simulink model "Cyber_Physical_Microgrid"  (R2024b)
settings: Solver=VariableStepAuto  StartTime=0.0  StopTime=270  RelTol=1e-3
values from neighbouring files (symbols this model uses):
  Bat =     [initData.mat]
  droopFC1 = 0.05    [initData.mat]
  droopFC2 = 0.05    [initData.mat]
  droopP2 = 0.05    [initData.mat]
  droopQ1 = 0.05    [initData.mat]
  droopQ2 = 0.05    [initData.mat]
  Pref2 = 0.8    [initData.mat]
  Qref1 = 0    [initData.mat]
  Qref2 = 0    [initData.mat]
  timeACLoadCurtail = 200    [initData.mat]
  timeSolarCurtail = 200    [initData.mat]
  Ts = 5e-05    [initData.mat]
  Ts_AC = 0.0002    [initData.mat]
  Ts_DC = 0.001    [initData.mat]
  volt2 = [270.467186401 250.166401688 246.278575679 243.847178474 242.073246789 240.654489675 239.457734124 238.414696845 237.485238449 236.643553985 235.871256975 235.151075236 ... (161 elements, 1x161)]    [initData.mat]
undefined symbols (not defined in the file or in its folder): BattTempBp, CapLUTBp, CapSOCBp, DiscIntNeverNeededParam, Em, Np, Ns, RInt, Tc_Batt
libraries: nesl_utility x55, fl_lib x52, ee_lib x39, modbuslib x16, spsRMSLib x8, simulink x5, spsFourierLib x2, batteryecm_lib x1, eeTransforms x1
(part 3 of 3)

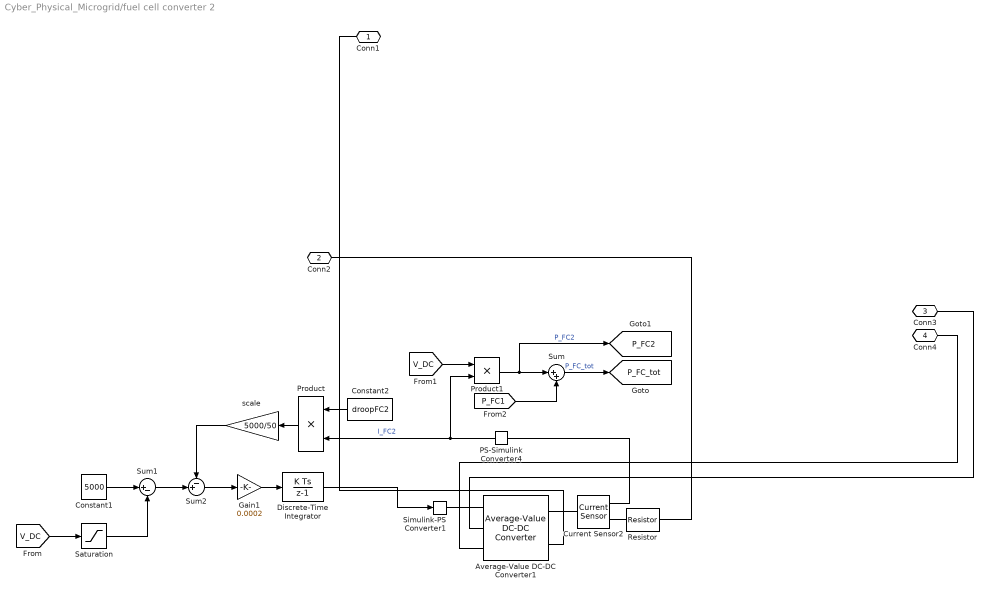
== system Cyber_Physical_Microgrid/fuel cell converter 2 ==
  Average-Value DC-DC Converter1 : ee_lib/Semiconductors & Converters/Converters/Average-Value DC-DC Converter  control_option=ee.enum.converters.controlinput.dutycycle  converter_type=ee.enum.converters.dcdctype.buckboost  efficiency_option=ee.enum.converters.efficiency.constant  efficiency_fixed=100  i_vec=[0, 2, 5] A  efficiency_vec=[90, 95, 98]
      settings: InternalSimscapePortConfiguration="{\"Bottom\":[],\"Left\":[{\"id\":\"DutyCycle\",\"label\":\"DutyCycle\",\"type\":\"input\"},{\"id\":\"p1\",\"label\":\"1+\",\"type\":\"foundation.electrical.electrical\"},{\"id\":\"n1\",\"label\":\"1-\",\"type\":\"foundation.electrical.electrical\"}],\"Right\":[{\"id\":\"p2\",\"label\":\"2+\",\"type\":\"foundation.electrical.electrical\"},{\"id\":\"n2\",\"label\":\"2-\",\"type\":\"foundation.electrical.electrical\"}],\"Top\":[]}"
  Constant1 : Constant  Value=5000  SampleTime=Ts_DC
  Constant2 : Constant  Value=droopFC2  SampleTime=Ts_DC
  Current Sensor2 : fl_lib/Electrical/Electrical Sensors/Current Sensor
  Discrete-Time Integrator : DiscreteIntegrator  InitialCondition=0.5  SampleTime=Ts_DC  LimitOutput=on  UpperSaturationLimit=0.99  LowerSaturationLimit=0  ICPrevOutput=DiscIntNeverNeededParam  ICPrevScaledInput=DiscIntNeverNeededParam
  Gain1 : Gain  Gain=0.0002
  PS-Simulink Converter4 : nesl_utility/PS-Simulink Converter  PhysicalDomain=network_engine_domain  SubClassName=ps_output  LeftPortType=input  RightPortType=output  PseudoPeriodic=off  Frequencies=[]  VectorFormat=1-D array  Unit=inherit  AffineConversion=off
  Product : Product
  Product1 : Product
  Resistor : fl_lib/Electrical/Electrical Elements/Resistor  R=1e-3 Ohm  i_specify=off  i_priority=None  i=0 A  i_nominal_specify=off  i_nominal_value=1  i_nominal_unit=A  v_specify=off  v_priority=None  v=0 V  v_nominal_specify=off  v_nominal_value=1  v_nominal_unit=V
  Saturation : Saturate  UpperLimit=5000
  Simulink-PS Converter1 : nesl_utility/Simulink-PS Converter  PhysicalDomain=network_engine_domain  SubClassName=ps_input  LeftPortType=input  RightPortType=output  PseudoPeriodic=off  Frequencies=[]  NoiseDistribution=none  NoiseParameters=[]  Unit=1  AffineConversion=off  FilteringAndDerivatives=provide  SimscapeFilterOrder=1  InputFilterTimeConstant=0.001  UdotUserProvided=0
  Sum : Sum  Inputs=|++
  Sum1 : Sum  Inputs=|+-
  Sum2 : Sum  Inputs=-+|
  scale : Gain  Gain=5000/50
  Conn1 : PMIOPort  Side=Right
  Conn2 : PMIOPort  Port=2  Side=Right
  Conn3 : PMIOPort  Port=3  Side=Left
  Conn4 : PMIOPort  Port=4  Side=Left
  tag scope: P_FC2=global, P_FC_tot=global
  wires:
  Sum/1 -> [P_FC_tot]  "P_FC_tot"
  Sum1/1 -> Sum2/2
  Product1/1 -> [P_FC2], Sum/1  "P_FC2"
  [P_FC1] -> Sum/2
  [V_DC] -> Product1/1
  Product/1 -> scale/1
  Discrete-Time Integrator/1 -> Simulink-PS Converter1/1
  Gain1/1 -> Discrete-Time Integrator/1
  PS-Simulink Converter4/1 -> Product/2, Product1/2  "I_FC2"
  scale/1 -> Sum2/1
  Constant2/1 -> Product/1
  Saturation/1 -> Sum1/2
  Sum2/1 -> Gain1/1
  Constant1/1 -> Sum1/1
  [V_DC] -> Saturation/1
  connections:
  Current Sensor2/RConn2 -- Resistor/LConn1
  Simulink-PS Converter1/RConn1 -- Average-Value DC-DC Converter1/LConn1
  Conn4/RConn1 -- Average-Value DC-DC Converter1/LConn3
  Conn3/RConn1 -- Average-Value DC-DC Converter1/LConn2
  Current Sensor2/LConn1 -- Average-Value DC-DC Converter1/RConn1
  PS-Simulink Converter4/LConn1 -- Current Sensor2/RConn1
  Average-Value DC-DC Converter1/RConn2 -- Conn1/RConn1
  Resistor/RConn1 -- Conn2/RConn1

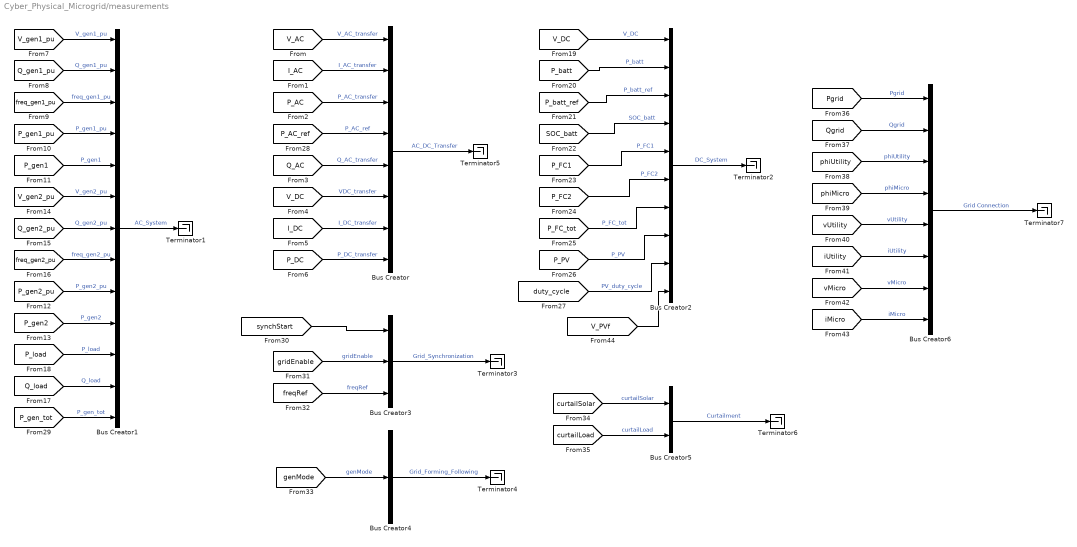
== system Cyber_Physical_Microgrid/measurements ==
  Bus Creator : BusCreator  Inputs=8
  Bus Creator1 : BusCreator  Inputs=13
  Bus Creator2 : BusCreator  Inputs=10
  Bus Creator3 : BusCreator  Inputs=3
  Bus Creator4 : BusCreator  Inputs=1
  Bus Creator5 : BusCreator  Inputs=2
  Bus Creator6 : BusCreator  Inputs=8
  Terminator{1..7} (7 alike) : Terminator
  wires:
  [V_AC] -> Bus Creator/1  "V_AC_transfer"
  [P_AC] -> Bus Creator/3  "P_AC_transfer"
  Bus Creator/1 -> Terminator5/1  "AC_DC_Transfer"
  [I_AC] -> Bus Creator/2  "I_AC_transfer"
  Bus Creator1/1 -> Terminator1/1  "AC_System"
  Bus Creator2/1 -> Terminator2/1  "DC_System"
  [V_gen1_pu] -> Bus Creator1/1  "V_gen1_pu"
  [Q_gen1_pu] -> Bus Creator1/2  "Q_gen1_pu"
  [freq_gen1_pu] -> Bus Creator1/3  "freq_gen1_pu"
  [P_gen1_pu] -> Bus Creator1/4  "P_gen1_pu"
  [P_gen1] -> Bus Creator1/5  "P_gen1"
  [V_gen2_pu] -> Bus Creator1/6  "V_gen2_pu"
  [Q_gen2_pu] -> Bus Creator1/7  "Q_gen2_pu"
  [freq_gen2_pu] -> Bus Creator1/8  "freq_gen2_pu"
  [P_gen2_pu] -> Bus Creator1/9  "P_gen2_pu"
  [P_gen2] -> Bus Creator1/10  "P_gen2"
  [P_load] -> Bus Creator1/11  "P_load"
  [Q_load] -> Bus Creator1/12  "Q_load"
  [V_DC] -> Bus Creator2/1  "V_DC"
  [P_batt] -> Bus Creator2/2  "P_batt"
  [P_batt_ref] -> Bus Creator2/3  "P_batt_ref"
  [SOC_batt] -> Bus Creator2/4  "SOC_batt"
  [P_FC1] -> Bus Creator2/5  "P_FC1"
  [P_FC2] -> Bus Creator2/6  "P_FC2"
  [P_FC_tot] -> Bus Creator2/7  "P_FC_tot"
  [P_PV] -> Bus Creator2/8  "P_PV"
  [duty_cycle] -> Bus Creator2/9  "PV_duty_cycle"
  [P_AC_ref] -> Bus Creator/4  "P_AC_ref"
  [Q_AC] -> Bus Creator/5  "Q_AC_transfer"
  [V_DC] -> Bus Creator/6  "VDC_transfer"
  [I_DC] -> Bus Creator/7  "I_DC_transfer"
  [P_DC] -> Bus Creator/8  "P_DC_transfer"
  [P_gen_tot] -> Bus Creator1/13  "P_gen_tot"
  [gridEnable] -> Bus Creator3/2  "gridEnable"
  Bus Creator3/1 -> Terminator3/1  "Grid_Synchronization"
  [freqRef] -> Bus Creator3/3  "freqRef"
  [genMode] -> Bus Creator4/1  "genMode"
  Bus Creator4/1 -> Terminator4/1  "Grid_Forming_Following"
  Bus Creator5/1 -> Terminator6/1  "Curtailment"
  [curtailLoad] -> Bus Creator5/2  "curtailLoad"
  [curtailSolar] -> Bus Creator5/1  "curtailSolar"
  [Pgrid] -> Bus Creator6/1  "Pgrid"
  [Qgrid] -> Bus Creator6/2  "Qgrid"
  Bus Creator6/1 -> Terminator7/1  "Grid Connection"
  [phiUtility] -> Bus Creator6/3  "phiUtility"
  [phiMicro] -> Bus Creator6/4  "phiMicro"
  [vUtility] -> Bus Creator6/5  "vUtility"
  [iUtility] -> Bus Creator6/6  "iUtility"
  [vMicro] -> Bus Creator6/7  "vMicro"
  [iMicro] -> Bus Creator6/8  "iMicro"
  [synchStart] -> Bus Creator3/1
  [V_PVf] -> Bus Creator2/10

== system Cyber_Physical_Microgrid/ /Form // Follow ==
  note: AVR and exciter control
  genMode : Inport
  Qerror : Inport  Port=2
  Verror : Inport  Port=3
  Constant1 : Constant  Value=500
  Constant2 : Constant  Value=0.5
  Constant3 : Constant  Value=1000
  Constant4 : Constant
  Discrete-Time Integrator : DiscreteIntegrator  gainval=1  InitialCondition=0.1  SampleTime=Ts_AC  ICPrevOutput=DiscIntNeverNeededParam  ICPrevScaledInput=DiscIntNeverNeededParam
  Product : Product
  Product1 : Product
  Sum4 : Sum  Inputs=|++
  Switch : Switch  Criteria=u2 > Threshold  SaturateOnIntegerOverflow=off  InputSameDT=off
  Switch1 : Switch  Criteria=u2 > Threshold  SaturateOnIntegerOverflow=off  InputSameDT=off
  Switch2 : Switch  Criteria=u2 > Threshold  SaturateOnIntegerOverflow=off  InputSameDT=off
  Unit Delay : UnitDelay  SampleTime=Ts_AC  HasFrameUpgradeWarning=on
  T : Outport
  wires:
  Product1/1 -> Unit Delay/1
  genMode/1 -> Switch/2, Switch2/2, Switch1/2
  Constant3/1 -> Switch2/3
  Constant4/1 -> Switch2/1
  Switch2/1 -> Product1/1
  Discrete-Time Integrator/1 -> Sum4/1
  Unit Delay/1 -> Sum4/2
  Constant2/1 -> Switch1/1
  Constant1/1 -> Switch1/3
  Switch/1 -> Product/2, Product1/2
  Product/1 -> Discrete-Time Integrator/1
  Verror/1 -> Switch/3
  Switch1/1 -> Product/1
  Qerror/1 -> Switch/1
  Sum4/1 -> T/1

== system Cyber_Physical_Microgrid/ /Form // Follow1 ==
  note: PRIME MOVER ND GOVRNR CONTROL
  genMode : Inport
  Perror : Inport  Port=2
  Ferror : Inport  Port=3
  Constant1 : Constant  Value=100
  Constant2 : Constant  Value=0.3
  Constant3 : Constant  Value=200
  Constant4 : Constant  Value=0.1
  Discrete-Time Integrator : DiscreteIntegrator  gainval=1  InitialCondition=0.1  SampleTime=Ts_AC  ICPrevOutput=DiscIntNeverNeededParam  ICPrevScaledInput=DiscIntNeverNeededParam
  Product : Product
  Product1 : Product
  Sum4 : Sum  Inputs=|++
  Switch : Switch  Criteria=u2 > Threshold  SaturateOnIntegerOverflow=off  InputSameDT=off
  Switch1 : Switch  Criteria=u2 > Threshold  SaturateOnIntegerOverflow=off  InputSameDT=off
  Switch2 : Switch  Criteria=u2 > Threshold  SaturateOnIntegerOverflow=off  InputSameDT=off
  Unit Delay : UnitDelay  SampleTime=Ts_AC  HasFrameUpgradeWarning=on
  T : Outport
  wires:
  Product1/1 -> Unit Delay/1
  genMode/1 -> Switch/2, Switch2/2, Switch1/2
  Constant3/1 -> Switch2/3
  Constant4/1 -> Switch2/1
  Switch2/1 -> Product1/1
  Discrete-Time Integrator/1 -> Sum4/1
  Unit Delay/1 -> Sum4/2
  Constant2/1 -> Switch1/1
  Constant1/1 -> Switch1/3
  Switch/1 -> Product/2, Product1/2
  Product/1 -> Discrete-Time Integrator/1
  Ferror/1 -> Switch/3
  Switch1/1 -> Product/1
  Perror/1 -> Switch/1
  Sum4/1 -> T/1

== system Cyber_Physical_Microgrid/Generator 02/Form // Follow ==
  genMode : Inport
  Qerror : Inport  Port=2
  Verror : Inport  Port=3
  Constant1 : Constant  Value=500
  Constant2 : Constant  Value=0.5
  Constant3 : Constant  Value=1000
  Constant4 : Constant
  Discrete-Time Integrator : DiscreteIntegrator  gainval=1  InitialCondition=0.1  SampleTime=Ts_AC  ICPrevOutput=DiscIntNeverNeededParam  ICPrevScaledInput=DiscIntNeverNeededParam
  Product : Product
  Product1 : Product
  Sum4 : Sum  Inputs=|++
  Switch : Switch  Criteria=u2 > Threshold  SaturateOnIntegerOverflow=off  InputSameDT=off
  Switch1 : Switch  Criteria=u2 > Threshold  SaturateOnIntegerOverflow=off  InputSameDT=off
  Switch2 : Switch  Criteria=u2 > Threshold  SaturateOnIntegerOverflow=off  InputSameDT=off
  Unit Delay : UnitDelay  SampleTime=Ts_AC  HasFrameUpgradeWarning=on
  T : Outport
  wires:
  Product1/1 -> Unit Delay/1
  genMode/1 -> Switch/2, Switch2/2, Switch1/2
  Constant3/1 -> Switch2/3
  Constant4/1 -> Switch2/1
  Switch2/1 -> Product1/1
  Discrete-Time Integrator/1 -> Sum4/1
  Unit Delay/1 -> Sum4/2
  Constant2/1 -> Switch1/1
  Constant1/1 -> Switch1/3
  Switch/1 -> Product/2, Product1/2
  Product/1 -> Discrete-Time Integrator/1
  Verror/1 -> Switch/3
  Switch1/1 -> Product/1
  Qerror/1 -> Switch/1
  Sum4/1 -> T/1

== system Cyber_Physical_Microgrid/Generator 02/Form // Follow1 ==
  genMode : Inport
  Perror : Inport  Port=2
  Ferror : Inport  Port=3
  Constant1 : Constant  Value=100
  Constant2 : Constant  Value=0.3
  Constant3 : Constant  Value=200
  Constant4 : Constant  Value=0.1
  Discrete-Time Integrator : DiscreteIntegrator  gainval=1  InitialCondition=0.1  SampleTime=Ts_AC  ICPrevOutput=DiscIntNeverNeededParam  ICPrevScaledInput=DiscIntNeverNeededParam
  Product : Product
  Product1 : Product
  Sum4 : Sum  Inputs=|++
  Switch : Switch  Criteria=u2 > Threshold  SaturateOnIntegerOverflow=off  InputSameDT=off
  Switch1 : Switch  Criteria=u2 > Threshold  SaturateOnIntegerOverflow=off  InputSameDT=off
  Switch2 : Switch  Criteria=u2 > Threshold  SaturateOnIntegerOverflow=off  InputSameDT=off
  Unit Delay : UnitDelay  SampleTime=Ts_AC  HasFrameUpgradeWarning=on
  T : Outport
  wires:
  Product1/1 -> Unit Delay/1
  genMode/1 -> Switch/2, Switch2/2, Switch1/2
  Constant3/1 -> Switch2/3
  Constant4/1 -> Switch2/1
  Switch2/1 -> Product1/1
  Discrete-Time Integrator/1 -> Sum4/1
  Unit Delay/1 -> Sum4/2
  Constant2/1 -> Switch1/1
  Constant1/1 -> Switch1/3
  Switch/1 -> Product1/2, Product/2
  Product/1 -> Discrete-Time Integrator/1
  Ferror/1 -> Switch/3
  Switch1/1 -> Product/1
  Perror/1 -> Switch/1
  Sum4/1 -> T/1

== system Cyber_Physical_Microgrid/Generator 02/Subsystem1 ==
  In1 : Inport
  Discrete-Time Integrator : DiscreteIntegrator  gainval=20  SampleTime=Ts_AC  ICPrevOutput=DiscIntNeverNeededParam  ICPrevScaledInput=DiscIntNeverNeededParam
  Sum : Sum  Inputs=|+-
  in1 : Outport
  wires:
  Sum/1 -> Discrete-Time Integrator/1
  Discrete-Time Integrator/1 -> Sum/2, in1/1
  In1/1 -> Sum/1

== system Cyber_Physical_Microgrid/Generator 02/Subsystem2 ==
  In1 : Inport
  Discrete-Time Integrator : DiscreteIntegrator  gainval=20  SampleTime=Ts_AC  ICPrevOutput=DiscIntNeverNeededParam  ICPrevScaledInput=DiscIntNeverNeededParam
  Sum : Sum  Inputs=|+-
  in : Outport
  wires:
  Sum/1 -> Discrete-Time Integrator/1
  Discrete-Time Integrator/1 -> Sum/2, in/1
  In1/1 -> Sum/1

== system Cyber_Physical_Microgrid/PQ meas/Subsystem ==
  In1 : Inport
  Discrete-Time Integrator : DiscreteIntegrator  gainval=20  SampleTime=Ts_AC  ICPrevOutput=DiscIntNeverNeededParam  ICPrevScaledInput=DiscIntNeverNeededParam
  Sum : Sum  Inputs=|+-
  Out1 : Outport
  wires:
  In1/1 -> Sum/1
  Discrete-Time Integrator/1 -> Out1/1, Sum/2
  Sum/1 -> Discrete-Time Integrator/1

== system Cyber_Physical_Microgrid/PQ meas/Subsystem1 ==
  In1 : Inport
  Discrete-Time Integrator : DiscreteIntegrator  gainval=20  SampleTime=Ts_AC  ICPrevOutput=DiscIntNeverNeededParam  ICPrevScaledInput=DiscIntNeverNeededParam
  Sum : Sum  Inputs=|+-
  Out1 : Outport
  wires:
  Sum/1 -> Discrete-Time Integrator/1
  Discrete-Time Integrator/1 -> Sum/2, Out1/1
  In1/1 -> Sum/1

== system Cyber_Physical_Microgrid/PV Array/Sensing Current ==
  Current Sensor : fl_lib/Electrical/Electrical Sensors/Current Sensor
  PS-Simulink/I : nesl_utility/PS-Simulink Converter  PhysicalDomain=network_engine_domain  SubClassName=ps_output  LeftPortType=input  RightPortType=output  PseudoPeriodic=off  Frequencies=[]  VectorFormat=1-D array  Unit=1  AffineConversion=off
  + : PMIOPort  Side=Left
  - : PMIOPort  Port=2  Side=Right
  I : Outport
  wires:
  PS-Simulink/I/1 -> I/1
  connections:
  -/RConn1 -- Current Sensor/RConn2
  Current Sensor/LConn1 -- +/RConn1
  Current Sensor/RConn1 -- PS-Simulink/I/LConn1

== system Cyber_Physical_Microgrid/PV Array/sensing voltage ==
  PS-Simulink Converter : nesl_utility/PS-Simulink Converter  PhysicalDomain=network_engine_domain  SubClassName=ps_output  LeftPortType=input  RightPortType=output  PseudoPeriodic=off  Frequencies=[]  VectorFormat=1-D array  Unit=inherit  AffineConversion=off
  Voltage Sensor : fl_lib/Electrical/Electrical Sensors/Voltage Sensor
  + : PMIOPort  Side=Left
  - : PMIOPort  Port=2  Side=Right
  V : Outport
  wires:
  PS-Simulink Converter/1 -> V/1
  connections:
  Voltage Sensor/LConn1 -- +/RConn1
  Voltage Sensor/RConn2 -- -/RConn1
  Voltage Sensor/RConn1 -- PS-Simulink Converter/LConn1

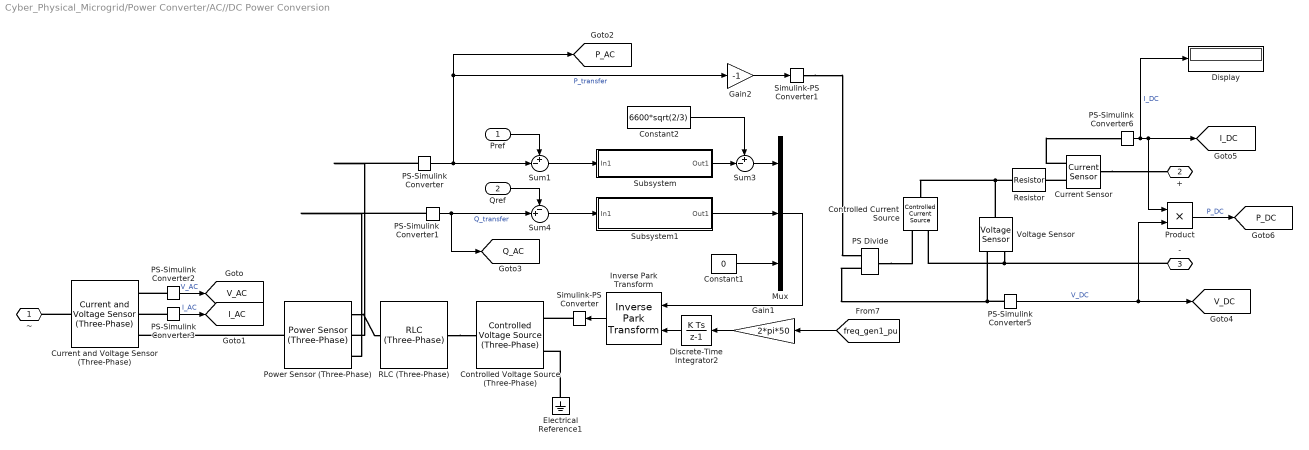
== system Cyber_Physical_Microgrid/Power Converter/AC//DC Power Conversion ==
  Pref : Inport
  Qref : Inport  Port=2
  Constant1 : Constant  Value=0
  Constant2 : Constant  Value=6600*sqrt(2/3)
  Controlled Current Source : fl_lib/Electrical/Electrical Sources/Controlled Current Source
  Controlled Voltage Source (Three-Phase) : ee_lib/Sources/Controlled Voltage Source (Three-Phase)  input_option=ee.enum.inputType.instantaneous  FRated=50 Hz
      settings: InternalSimscapePortConfiguration="{\"Bottom\":[],\"Left\":[{\"id\":\"S\",\"label\":\"S\",\"type\":\"input\"},{\"id\":\"n\",\"label\":\"n\",\"type\":\"foundation.electrical.electrical\"}],\"Right\":[{\"id\":\"N\",\"label\":\"~\",\"type\":\"foundation.electrical.three_phase\"}],\"Top\":[]}"
  Current Sensor : fl_lib/Electrical/Electrical Sensors/Current Sensor
  Current and Voltage Sensor (Three-Phase) : ee_lib/Sensors & Transducers/Current and Voltage Sensor (Three-Phase)  vMeasurementType=ee.enum.vmeasurement.ll  outputUnit=ee.enum.unit.si  SRated=100e6 A*V  VRated=24e3 V  I_specify=off  I_priority=None  I=[0, 0, 0] A  I_nominal_specify=off  I_nominal_value=1  I_nominal_unit=A  V_specify=off  V_priority=None  V=[0, 0, 0] V  V_nominal_specify=off  V_nominal_value=1  V_nominal_unit=V
      settings: InternalSimscapePortConfiguration="{\"Bottom\":[],\"Left\":[{\"id\":\"N1\",\"label\":\"~1\",\"type\":\"foundation.electrical.three_phase\"}],\"Right\":[{\"id\":\"V_output\",\"label\":\"V\",\"type\":\"output\"},{\"id\":\"I_output\",\"label\":\"I\",\"type\":\"output\"},{\"id\":\"N2\",\"label\":\"~2\",\"type\":\"foundation.electrical.three_phase\"}],\"Top\":[]}"
  Discrete-Time Integrator2 : DiscreteIntegrator  SampleTime=Ts_AC  ICPrevOutput=DiscIntNeverNeededParam  ICPrevScaledInput=DiscIntNeverNeededParam
  Display : Display
  Electrical Reference1 : fl_lib/Electrical/Electrical Elements/Electrical Reference
  Gain1 : Gain  Gain=2*pi*50
  Gain2 : Gain  Gain=-1
  Inverse Park Transform : eeTransforms/Inverse Park Transform  AxisAlignment=Q-axis  PowerInvariant=off
  Mux : Mux  Inputs=3
  PS Divide : fl_lib/Physical Signals/Functions/PS Divide
  PS-Simulink Converter : nesl_utility/PS-Simulink Converter  PhysicalDomain=network_engine_domain  SubClassName=ps_output  LeftPortType=input  RightPortType=output  PseudoPeriodic=off  Frequencies=[]  VectorFormat=1-D array  Unit=W  AffineConversion=off
  PS-Simulink Converter1 : nesl_utility/PS-Simulink Converter  PhysicalDomain=network_engine_domain  SubClassName=ps_output  LeftPortType=input  RightPortType=output  PseudoPeriodic=off  Frequencies=[]  VectorFormat=1-D array  Unit=V*A  AffineConversion=off
  PS-Simulink Converter{2..3,5..6} (4 alike) : nesl_utility/PS-Simulink Converter  PhysicalDomain=network_engine_domain  SubClassName=ps_output  LeftPortType=input  RightPortType=output  PseudoPeriodic=off  Frequencies=[]  VectorFormat=1-D array  Unit=inherit  AffineConversion=off
  Power Sensor (Three-Phase) : ee_lib/Sensors & Transducers/Power Sensor (Three-Phase)  load_type=ee.enum.passive.type_balanced.balanced  f0=50 Hz
      settings: InternalSimscapePortConfiguration="{\"Bottom\":[],\"Left\":[{\"id\":\"N1\",\"label\":\"~1\",\"type\":\"foundation.electrical.three_phase\"}],\"Right\":[{\"id\":\"N2\",\"label\":\"~2\",\"type\":\"foundation.electrical.three_phase\"}],\"Top\":[{\"id\":\"Pm\",\"label\":\"P\",\"type\":\"output\"},{\"id\":\"Qm\",\"label\":\"Q\",\"type\":\"output\"}]}"
  Product : Product
  RLC (Three-Phase) : ee_lib/Passive/RLC Assemblies/RLC (Three-Phase)  port_option=ee.enum.threePhasePort.composite  component_structure=ee.enum.rlc.structure.L  R=1e-2 Ohm  L=5e-2 H  C=1e-6 F  R_parasitic=1e-6 Ohm  G_parasitic=0 1/Ohm  IL_specify=off  IL_priority=High  IL=[0, 0, 0] A  IL_nominal_specify=off  IL_nominal_value=1  IL_nominal_unit=A  VC_specify=off  VC_priority=High  VC=[0, 0, 0] V  VC_nominal_specify=off  VC_nominal_value=1  VC_nominal_unit=V
      settings: InternalSimscapePortConfiguration="{\"Bottom\":[],\"Left\":[{\"id\":\"N1\",\"label\":\"~1\",\"type\":\"foundation.electrical.three_phase\"}],\"Right\":[{\"id\":\"N2\",\"label\":\"~2\",\"type\":\"foundation.electrical.three_phase\"}],\"Top\":[]}"
  Resistor : fl_lib/Electrical/Electrical Elements/Resistor  R=1e-3 Ohm  i_specify=off  i_priority=None  i=0 A  i_nominal_specify=off  i_nominal_value=1  i_nominal_unit=A  v_specify=off  v_priority=None  v=0 V  v_nominal_specify=off  v_nominal_value=1  v_nominal_unit=V
  Simulink-PS Converter : nesl_utility/Simulink-PS Converter  PhysicalDomain=network_engine_domain  SubClassName=ps_input  LeftPortType=input  RightPortType=output  PseudoPeriodic=off  Frequencies=[]  NoiseDistribution=none  NoiseParameters=[]  Unit=1  AffineConversion=off  FilteringAndDerivatives=provide  SimscapeFilterOrder=1  InputFilterTimeConstant=0.001  UdotUserProvided=0
  Simulink-PS Converter1 : nesl_utility/Simulink-PS Converter  PhysicalDomain=network_engine_domain  SubClassName=ps_input  LeftPortType=input  RightPortType=output  PseudoPeriodic=off  Frequencies=[]  NoiseDistribution=none  NoiseParameters=[]  Unit=W  AffineConversion=off  FilteringAndDerivatives=provide  SimscapeFilterOrder=1  InputFilterTimeConstant=0.001  UdotUserProvided=0
  Subsystem : Subsystem
      mask Display: disp('Active Power Control')
  Subsystem1 : Subsystem
      mask Display: disp('Reactive Power Control')
  Sum1 : Sum  Inputs=+-|
  Sum3 : Sum  Inputs=+-|
  Sum4 : Sum  Inputs=-+|
  Voltage Sensor : fl_lib/Electrical/Electrical Sensors/Voltage Sensor
  ~ : PMIOPort  Side=Left
  + : PMIOPort  Port=2  Side=Right
  - : PMIOPort  Port=3  Side=Right
  tag scope: I_AC=global, I_DC=global, P_AC=global, P_DC=global, Q_AC=global, V_AC=global, V_DC=global
  wires:
  PS-Simulink Converter1/1 -> [Q_AC], Sum4/2  "Q_transfer"
  Constant1/1 -> Mux/3
  Sum4/1 -> Subsystem1/1(In1)
  Sum1/1 -> Subsystem/1(In1)
  Qref/1 -> Sum4/1
  Inverse Park Transform/1 -> Simulink-PS Converter/1
  Sum3/1 -> Mux/1
  Discrete-Time Integrator2/1 -> Inverse Park Transform/2
  Pref/1 -> Sum1/1
  PS-Simulink Converter3/1 -> [I_AC]  "I_AC"
  PS-Simulink Converter2/1 -> [V_AC]  "V_AC"
  Mux/1 -> Inverse Park Transform/1
  Constant2/1 -> Sum3/1
  Gain1/1 -> Discrete-Time Integrator2/1
  Subsystem1/1(Out1) -> Mux/2
  Subsystem/1(Out1) -> Sum3/2
  [freq_gen1_pu] -> Gain1/1
  PS-Simulink Converter6/1 -> Display/1, [I_DC], Product/1  "I_DC"
  PS-Simulink Converter5/1 -> [V_DC], Product/2  "V_DC"
  Product/1 -> [P_DC]  "P_DC"
  PS-Simulink Converter/1 -> [P_AC], Gain2/1, Sum1/2  "P_transfer"
  Gain2/1 -> Simulink-PS Converter1/1
  connections:
  Electrical Reference1/LConn1 -- Controlled Voltage Source (Three-Phase)/LConn2
  Simulink-PS Converter/RConn1 -- Controlled Voltage Source (Three-Phase)/LConn1
  PS-Simulink Converter1/LConn1 -- Power Sensor (Three-Phase)/LConn3
  PS-Simulink Converter/LConn1 -- Power Sensor (Three-Phase)/LConn2
  PS-Simulink Converter2/LConn1 -- Current and Voltage Sensor (Three-Phase)/RConn1
  PS-Simulink Converter3/LConn1 -- Current and Voltage Sensor (Three-Phase)/RConn2
  Current and Voltage Sensor (Three-Phase)/LConn1 -- ~/RConn1
  RLC (Three-Phase)/RConn1 -- Controlled Voltage Source (Three-Phase)/RConn1
  PS-Simulink Converter5/LConn1 -- PS Divide/LConn2 -- Voltage Sensor/RConn1
  Voltage Sensor/RConn2 -- Controlled Current Source/RConn2 -- -/RConn1
  Resistor/LConn1 -- Controlled Current Source/LConn1 -- Voltage Sensor/LConn1
  Current Sensor/RConn2 -- Resistor/RConn1
  Simulink-PS Converter1/RConn1 -- PS Divide/LConn1
  Current Sensor/RConn1 -- PS-Simulink Converter6/LConn1
  Current Sensor/LConn1 -- +/RConn1
  PS Divide/RConn1 -- Controlled Current Source/RConn1
  Power Sensor (Three-Phase)/RConn1 -- Current and Voltage Sensor (Three-Phase)/RConn3
  Power Sensor (Three-Phase)/LConn1 -- RLC (Three-Phase)/LConn1

== system Cyber_Physical_Microgrid/Power Converter/AC//DC Power Conversion/Subsystem ==
  note: Active power control
  In1 : Inport
  Discrete-Time Integrator1 : DiscreteIntegrator  gainval=1  SampleTime=Ts_AC  ICPrevOutput=DiscIntNeverNeededParam  ICPrevScaledInput=DiscIntNeverNeededParam
  Gain : Gain  Gain=-2e-3*50
  Gain1 : Gain  Gain=-2e-3
  Scope : Scope
  Sum2 : Sum  Inputs=|++
  Unit Delay : UnitDelay  SampleTime=Ts_AC  HasFrameUpgradeWarning=on
  Out1 : Outport
  wires:
  In1/1 -> Gain/1, Gain1/1
  Gain1/1 -> Unit Delay/1
  Gain/1 -> Discrete-Time Integrator1/1
  Sum2/1 -> Scope/1, Out1/1
  Discrete-Time Integrator1/1 -> Sum2/1
  Unit Delay/1 -> Sum2/2

== system Cyber_Physical_Microgrid/Power Converter/AC//DC Power Conversion/Subsystem1 ==
  note: Reactive power control
  In1 : Inport
  Discrete-Time Integrator3 : DiscreteIntegrator  gainval=1  SampleTime=Ts_AC  ICPrevOutput=DiscIntNeverNeededParam  ICPrevScaledInput=DiscIntNeverNeededParam
  Gain2 : Gain  Gain=1e-3*500
  Gain3 : Gain  Gain=1e-4*100
  Sum5 : Sum  Inputs=|++
  Unit Delay1 : UnitDelay  SampleTime=Ts_AC  HasFrameUpgradeWarning=on
  Out1 : Outport
  wires:
  Gain2/1 -> Discrete-Time Integrator3/1
  Sum5/1 -> Out1/1
  Unit Delay1/1 -> Sum5/2
  Gain3/1 -> Unit Delay1/1
  Discrete-Time Integrator3/1 -> Sum5/1
  In1/1 -> Gain2/1, Gain3/1

== matlab function Cyber_Physical_Microgrid/Grid Synchronization/Grid Synchronization1 ==
  data: deltaF input; freqUtility input; freqMicro input; freqRef output; phiUtility input; phiMicro input; gridEnable output; synchStart input
function [freqRef,gridEnable] = gridSynchronization(deltaF,freqUtility,freqMicro,phiUtility,phiMicro,synchStart)

persistent freqRefold gridEnableold

if isempty(freqRefold)
 
    freqRefold = 1;

    gridEnableold = 1; % 1 means we are islanded, 0 means we are connected to the utility grid
 
end

dF = freqUtility - freqMicro; % frequency delta between utility grid and microgrid

if abs(dF) > 1e-4 && synchStart == 1 && gridEnableold == 1 % frequency is not within tolerance

    if dF < 0 % adjust frequency setpoint incrementally

        freqRef = freqRefold - deltaF;

    else

        freqRef = freqRefold + deltaF;

    end

    gridEnableold = 1;
    
elseif abs(dF) < 1e-4 && synchStart == 1 && gridEnableold == 1 % frequency is within tolerance

    if abs(phiUtility - phiMicro) < 1e-2  % wait for phase to be within tolerance

        gridEnableold = 0;

    else
 
        gridEnableold = 1;

    end

    freqRef = freqRefold;

    
elseif synchStart == 0 % if we do not have an active synchronization signal, stay islanded

    freqRef = freqRefold;

    gridEnableold = 1;

else % grid connection is enabled

    freqRef = freqRefold;

    gridEnableold = 0;

end

freqRefold = freqRef;

gridEnable = gridEnableold;

== matlab function Cyber_Physical_Microgrid/Grid Forming Following/Grid Forming // Grid Following ==
  data: gridEnable input; genMode output
function genMode = gridFormingFollowing(gridEnable)

if gridEnable == 1 % grid forming

    genMode = 0;

else % grid following

    genMode = 1; 

end

== matlab function Cyber_Physical_Microgrid/Generator 02/MATLAB Function1 ==
  data: in1 input; droopP2 output; alpha1 input
function droopP2 = DroopP2(in1, alpha1)
%#codegen
droopP2 = in1 .* alpha1;
end

== matlab function Cyber_Physical_Microgrid/Generator 02/MATLAB Function ==
  data: in1 input; droopQ2 output; alpha1 input
function droopQ2 = DroopQ2(in1, alpha1)
%#codegen
droopQ2 = in1 .* alpha1;
end

== matlab function Cyber_Physical_Microgrid/PV converter/MPPT Controller using Pertrb & Obsere technque  ==
  settings: updateMethod=DISCRETE  sampleTime=Ts_DC
  data: Param input; Enabled input; V input; I input; D output
function D  = controller(Param, Enabled, V, I)

% MPPT controller based on the Perturb & Observe algorithm.

% D output = Duty cycle of the boost converter (value between 0 and 1)
%
% Enabled input = 1 to enable the MPPT controller
% V input = PV array terminal voltage (V)
% I input = PV array current (A)
%
% Param input:
Dinit = Param(1);  %Initial value for D output
Dmax = Param(2);   %Maximum value for D
Dmin = Param(3);   %Minimum value for D
deltaD = Param(4); %Increment value used to increase/decrease the duty cycle D
% ( increasing D = decreasing Vref )
%  

persistent Vold Pold Dold;

dataType = 'double';

if isempty(Vold)
    Vold=0;
    Pold=0;
    Dold=Dinit;
end
P= V*I;
dV= V - Vold;
dP= P - Pold;

 if dP ~= 0 & Enabled ~=0
%     if dP>1e-9  & dP<-1e-9 & Enabled ~=0
    if dP < 0
        if dV < 0
            D = Dold - deltaD;
        else
            D = Dold + deltaD;
        end
    else
        if dV < 0
            D = Dold + deltaD;
        else
            D = Dold - deltaD;
        end    
    end
else D=Dold;
end

if D >= Dmax | D<= Dmin
    D=Dold;
end

Dold=D;
Vold=V;
Pold=P;
